simulink model "PIDmodel_nsat"  (R2015a)
settings: Solver=ode45  StartTime=0.0  StopTime=simulation_time  FixedStep=sim_step  RelTol=1e-3
undefined symbols (not defined in the file or in its folder): ctr, K_i, K_p
libraries: cstblocks x1, simulink x1
settings Model: Creator=wk  LastModifiedBy=Milosz
settings DebuggingCC: UnderspecifiedInitializationDetection=Classic  MergeDetectMultiDrivingBlocksExec=none  StateNameClashWarn=warning

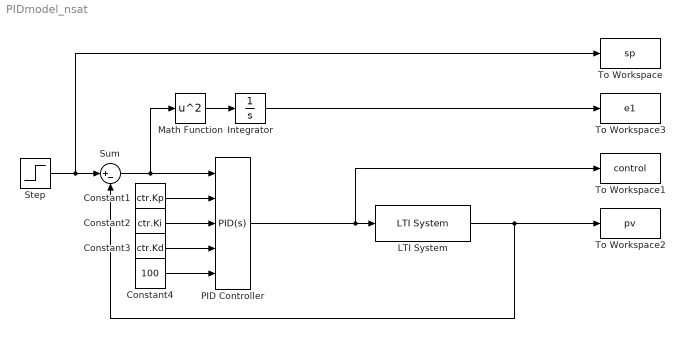
== system PIDmodel_nsat ==
  Constant1 : Constant  Value=ctr.Kp
  Constant2 : Constant  Value=ctr.Ki
  Constant3 : Constant  Value=ctr.Kd
  Constant4 : Constant  Value=100
  Integrator : Integrator
  LTI System : cstblocks/LTI System  sys=G  IC=[]
  Math Function : Math  Operator=square  SaturateOnIntegerOverflow=on
  PID Controller : simulink/Continuous/PID Controller  Controller=PID  TimeDomain=Continuous-time  SampleTime=-1  IntegratorMethod=Forward Euler  FilterMethod=Forward Euler  Form=Parallel  UseFilter=on  ControllerParametersSource=external  P=K_p  I=K_i  D=0  N=100  InitialConditionSource=internal  InitialConditionForIntegrator=0  InitialConditionForFilter=0  ExternalReset=none  LimitOutput=off  UpperSaturationLimit=inf  LowerSaturationLimit=-inf  LinearizeAsGain=on  AntiWindupMode=none  Kb=1  TrackingMode=off  Kt=1  PParamMin=[]  PParamMax=[]  IParamMin=[]  IParamMax=[]  DParamMin=[]  DParamMax=[]  NParamMin=[]  NParamMax=[]  KbParamMin=[]  KbParamMax=[]  KtParamMin=[]  KtParamMax=[]  POutMin=[]  POutMax=[]  IOutMin=[]  IOutMax=[]  DOutMin=[]  DOutMax=[]  NOutMin=[]  NOutMax=[]  KbOutMin=[]  KbOutMax=[]  KtOutMin=[]  KtOutMax=[]  IntegratorOutMin=[]  IntegratorOutMax=[]  FilterOutMin=[]  FilterOutMax=[]  SumOutMin=[]  SumOutMax=[]  SumI1OutMin=[]  SumI1OutMax=[]  SumI2OutMin=[]  SumI2OutMax=[]  SumI3OutMin=[]  SumI3OutMax=[]  SumDOutMin=[]  SumDOutMax=[]  SaturationOutMin=[]  SaturationOutMax=[]  IntegratorContinuousStateAttributes=''  IntegratorStateMustResolveToSignalObject=off  IntegratorRTWStateStorageClass=Auto  FilterContinuousStateAttributes=''  FilterStateMustResolveToSignalObject=off  FilterRTWStateStorageClass=Auto  DifferentiatorICPrevScaledInput=0  DifferentiatorOutMin=[]  DifferentiatorOutMax=[]
  Step : Step  SampleTime=0
  Sum : Sum  Inputs=|+-
  To Workspace : ToWorkspace  VariableName=sp  SaveFormat=Timeseries  SampleTime=-1
  To Workspace1 : ToWorkspace  VariableName=control  SaveFormat=Timeseries  SampleTime=-1
  To Workspace2 : ToWorkspace  VariableName=pv  SaveFormat=Timeseries  SampleTime=-1
  To Workspace3 : ToWorkspace  VariableName=e1  SaveFormat=Timeseries  SampleTime=-1
  wires:
  Step/1 -> To Workspace/1, Sum/1
  Sum/1 -> Math Function/1, PID Controller/1
  LTI System/1 -> Sum/2, To Workspace2/1
  Constant4/1 -> PID Controller/5
  Constant3/1 -> PID Controller/4
  Constant2/1 -> PID Controller/3
  Constant1/1 -> PID Controller/2
  PID Controller/1 -> To Workspace1/1, LTI System/1
  Math Function/1 -> Integrator/1
  Integrator/1 -> To Workspace3/1
